simulink model "main"  (R2017a)
settings: Solver=VariableStepAuto  StartTime=0.0  StopTime=10.0  RelTol=1e-3
settings Model: Creator=eduardo  LastModifiedBy=eduardo

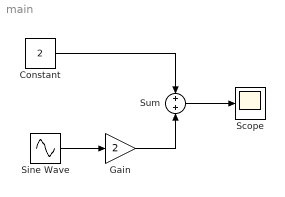
== system main ==
  Constant : Constant  Value=2
  Gain : Gain  Gain=2
  Scope : Scope
  Sine Wave : Sin  SampleTime=0
  Sum : Sum  Inputs=+|+
  wires:
  Sine Wave/1 -> Gain/1
  Sum/1 -> Scope/1
  Constant/1 -> Sum/1
  Gain/1 -> Sum/2
